simulink model "camara_termicaprofwilkley_editado_2507"  (R2022a)
settings: Solver=VariableStepAuto  StartTime=0.0  StopTime=400  RelTol=1e-3
values from neighbouring files (symbols this model uses):
  Ha = Hss.A    [Camara_Termica.m]
  Hb = Hss.B    [Camara_Termica.m]
  Hc = Hss.C    [Camara_Termica.m]
  K1 = Klinha(1,5)    [Camara_Termica.m]
  K2 = Klinha(3,5)    [Camara_Termica.m]
  K3 = Klinha(6,5)    [Camara_Termica.m]
  K4 = Klinha(6,6)    [Camara_Termica.m]
  Kx = Klinha(1:4,1:4)    [Camara_Termica.m]
settings Model: Creator=CARLOS HOLANDA  LastModifiedBy=CARLOS HOLANDA
settings DebuggingCC: UnconnectedInputMsg=warning  UnconnectedOutputMsg=warning  UnconnectedLineMsg=warning
settings RTWCC: DLArmComputeVersion=19.05

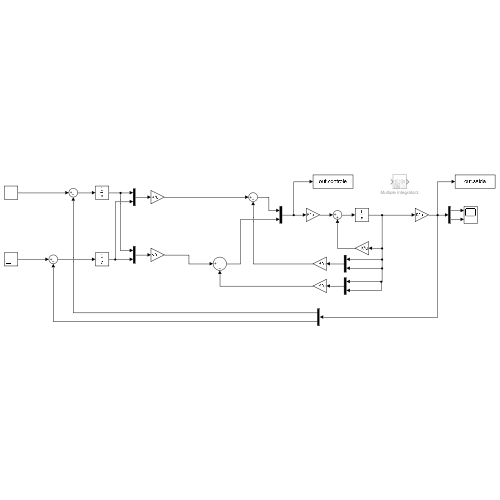
[thumbnail: Simulink's stored preview of the top-level diagram]
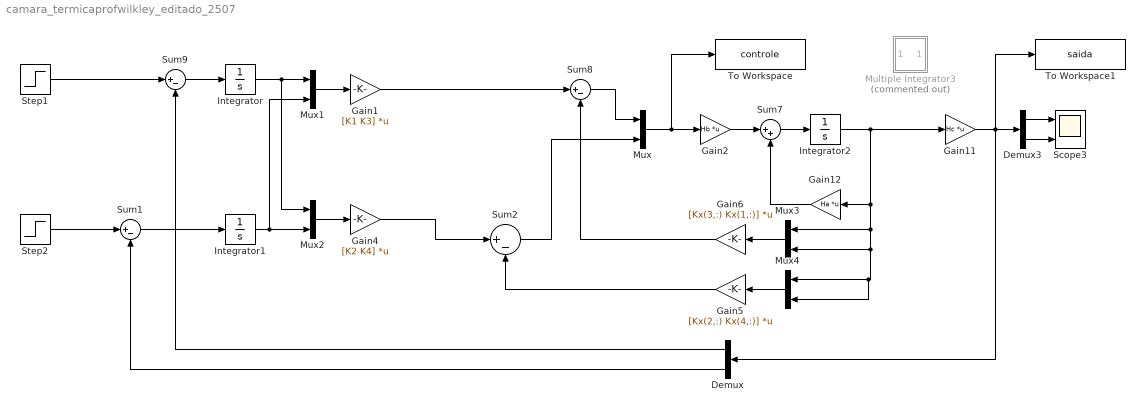
== system camara_termicaprofwilkley_editado_2507 ==
  Demux : Demux  Outputs=2
  Demux3 : Demux  Outputs=2
  Gain1 : Gain  Gain=[K1 K3]  Multiplication=Matrix(K*u)
  Gain11 : Gain  Gain=Hc  Multiplication=Matrix(K*u)
  Gain12 : Gain  Gain=Ha  Multiplication=Matrix(K*u)
  Gain2 : Gain  Gain=Hb  Multiplication=Matrix(K*u)
  Gain4 : Gain  Gain=[K2 K4]  Multiplication=Matrix(K*u)
  Gain5 : Gain  Gain=[Kx(2,:) Kx(4,:)]  Multiplication=Matrix(K*u)
  Gain6 : Gain  Gain=[Kx(3,:) Kx(1,:)]  Multiplication=Matrix(K*u)
  Integrator : Integrator
  Integrator1 : Integrator
  Integrator2 : Integrator
  Multiple Integrator3 : Subsystem  Commented=on
  Mux{,1..4} (5 alike) : Mux  Inputs=2
  Scope3 : Scope  NumInputPorts=2
  Step1 : Step  Time=0  After=-3  SampleTime=0
  Step2 : Step  Time=200  After=2  SampleTime=0
  Sum{1..2,8..9} (4 alike) : Sum  Inputs=|+-
  Sum7 : Sum  Inputs=|++
  To Workspace : ToWorkspace  VariableName=controle  SaveFormat=Timeseries  SampleTime=-1
  To Workspace1 : ToWorkspace  VariableName=saida  SaveFormat=Timeseries  SampleTime=-1
  wires:
  Step1/1 -> Sum9/1
  Demux3/1 -> Scope3/1
  Gain12/1 -> Sum7/2
  Gain11/1 -> To Workspace1/1, Demux/1, Demux3/1
  Sum7/1 -> Integrator2/1
  Demux3/2 -> Scope3/2
  Integrator2/1 -> Mux3/1, Mux4/2, Mux4/1, Mux3/2, Gain12/1, Gain11/1
  Sum9/1 -> Integrator/1
  Gain2/1 -> Sum7/1
  Demux/1 -> Sum9/2
  Demux/2 -> Sum1/2
  Step2/1 -> Sum1/1
  Integrator1/1 -> Mux2/2, Mux1/2
  Sum1/1 -> Integrator1/1
  Sum8/1 -> Mux/1
  Sum2/1 -> Mux/2
  Mux/1 -> To Workspace/1, Gain2/1
  Gain6/1 -> Sum8/2
  Gain5/1 -> Sum2/2
  Gain1/1 -> Sum8/1
  Integrator/1 -> Mux2/1, Mux1/1
  Mux1/1 -> Gain1/1
  Mux2/1 -> Gain4/1
  Gain4/1 -> Sum2/1
  Mux3/1 -> Gain6/1
  Mux4/1 -> Gain5/1

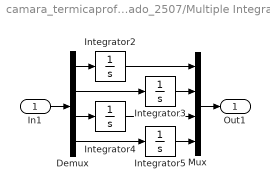
== system camara_termicaprofwilkley_editado_2507/Multiple Integrator3 ==
  In1 : Inport
  Demux : Demux
  Integrator{2..5} (4 alike) : Integrator
  Mux : Mux
  Out1 : Outport
  wires:
  Mux/1 -> Out1/1
  Integrator2/1 -> Mux/1
  Demux/3 -> Integrator4/1
  Demux/4 -> Integrator5/1
  Demux/2 -> Integrator3/1
  Integrator4/1 -> Mux/3
  Integrator3/1 -> Mux/2
  Integrator5/1 -> Mux/4
  Demux/1 -> Integrator2/1
  In1/1 -> Demux/1
